simulink model "ex_04_model"  (R2014a)
settings: Solver=ode45  StartTime=0.0  StopTime=10.0  RelTol=1e-3
undefined symbols (not defined in the file): G, x, y, z
settings Model: Creator=Nino  LastModifiedBy=Nino

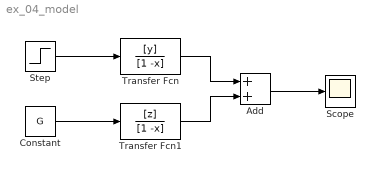
== system ex_04_model ==
  Add : Sum
  Constant : Constant  Value=G
  Scope : Scope
  Step : Step  After=10  SampleTime=0
  Transfer Fcn : TransferFcn  Numerator=[y]  Denominator=[1 -x]
  Transfer Fcn1 : TransferFcn  Numerator=[z]  Denominator=[1 -x]
  wires:
  Transfer Fcn/1 -> Add/1
  Transfer Fcn1/1 -> Add/2
  Add/1 -> Scope/1
  Step/1 -> Transfer Fcn/1
  Constant/1 -> Transfer Fcn1/1
